simulink model "MAIN"  (R2023a)
settings: Solver=FixedStepDiscrete  StartTime=0.0  StopTime=10.0  FixedStep=1e-5  RelTol=1e-3
libraries: eeGeneralControl x2, simulink_extras x1
settings Model: Creator=james  LastModifiedBy=james
settings OptimizationCC: DefaultParameterBehavior=Inlined  UseDivisionForNetSlopeComputation=on  GainParamInheritBuiltInType=on  UseFloatMulNetSlope=on  InlineInvariantSignals=on  PassReuseOutputArgsAs=Individual arguments  ZeroExternalMemoryAtStartup=off  ZeroInternalMemoryAtStartup=off  NoFixptDivByZeroProtection=on  EfficientFloat2IntCast=on  LifeSpan=1  OptimizeBlockOrder=speed  DifferentSizesBufferReuse=on  EfficientTunableParamExpr=on
settings DebuggingCC: ParameterTunabilityLossMsg=error
settings HardwareCC: ProdBitPerPointer=32  ProdBitPerSizeT=32  ProdBitPerPtrDiffT=32  ProdLargestAtomicInteger=Long  ProdLargestAtomicFloat=Double  ProdWordSize=32  ProdLongLongMode=on  ProdHWDeviceType=ARM Compatible->ARM Cortex-M
settings SFSimCC: MATLABDynamicMemAlloc=off
settings RTWCC: Description=Embedded Coder  SystemTargetFile=ert.tlc  GenCodeOnly=on  TemplateMakefile=ert_default_tmf  GenerateReport=on  LaunchReport=on  GenerateCodeReplacementReport=on
settings CodeAppCC: ForceParamTrailComments=on  IgnoreCustomStorageClasses=off  OperatorAnnotations=on  SimulinkDataObjDesc=on  SFDataObjDesc=on  CustomSymbolStrGlobalVar=rt$N$M  CustomSymbolStrType=$N$M  CustomSymbolStrFcn=$N$M$F  CustomSymbolStrMacro=$N$M  InsertBlockDesc=on
settings ERTTargetCC: TargetLangStandard=C99 (ISO)  CodeReplacementLibrary=ARM Cortex-M  GenerateSampleERTMain=on  IncludeMdlTerminateFcn=off  CombineSignalStateStructs=on  SuppressErrorStatus=on  SupportAbsoluteTime=off  SupportNonFinite=off  SupportComplex=off  InlinedParameterPlacement=NonHierarchical  ERTCustomFileTemplate=example_file_process.tlc  ERTFilePackagingFormat=CompactWithDataFile

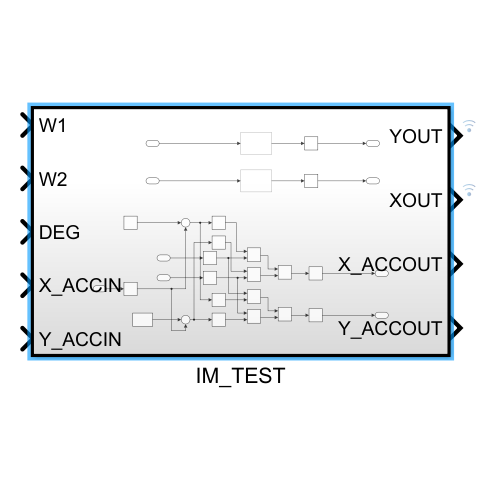
[thumbnail: Simulink's stored preview of the top-level diagram]
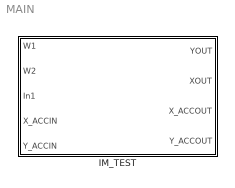
== system MAIN ==
  IM_TEST : Subsystem  TreatAsAtomicUnit=on
      settings: RTWSystemCode=Nonreusable function

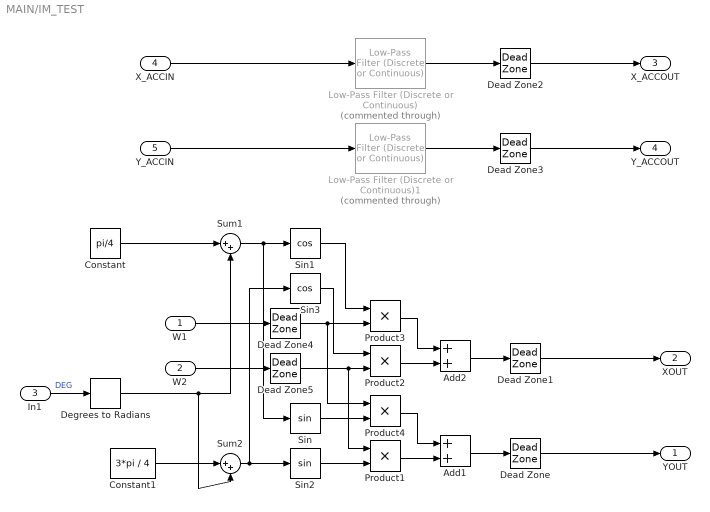
== system MAIN/IM_TEST ==
  W1 : Inport  OutDataTypeStr=single  LockScale=on
  W2 : Inport  Port=2  OutDataTypeStr=single  LockScale=on
  In1 : Inport  Port=3  OutDataTypeStr=single
  X_ACCIN : Inport  Port=4
  Y_ACCIN : Inport  Port=5
  Add1 : Sum
  Add2 : Sum
  Constant : Constant  Value=pi/4  OutDataTypeStr=single  LockScale=on
  Constant1 : Constant  Value=3*pi / 4  OutDataTypeStr=single  LockScale=on
  Dead Zone : DeadZone  LowerValue=-0.0005  UpperValue=0.00005
  Dead Zone1 : DeadZone  LowerValue=-0.0005  UpperValue=0.00005
  Dead Zone2 : DeadZone  LowerValue=-0.1  UpperValue=0.1
  Dead Zone3 : DeadZone  LowerValue=-0.1  UpperValue=0.1
  Dead Zone4 : DeadZone  LowerValue=-30  UpperValue=30
  Dead Zone5 : DeadZone  LowerValue=-30  UpperValue=30
  Degrees to Radians : simulink_extras/Transformations/Degrees to Radians
  Low-Pass Filter (Discrete or Continuous) : eeGeneralControl/Low-Pass Filter (Discrete or Continuous)  Commented=through  K=1  T=0.1  B=inf  A=-inf  init_option=Inherited from block input  x0=0  Ts=-1
  Low-Pass Filter (Discrete or Continuous)1 : eeGeneralControl/Low-Pass Filter (Discrete or Continuous)  Commented=through  K=1  T=0.1  B=inf  A=-inf  init_option=Inherited from block input  x0=0  Ts=-1
  Product{1..4} (4 alike) : Product
  Sin : Trigonometry  ApproximationMethod=Lookup
  Sin1 : Trigonometry  Operator=cos  ApproximationMethod=Lookup
  Sin2 : Trigonometry  ApproximationMethod=Lookup  OutputSignalType=real
  Sin3 : Trigonometry  Operator=cos  ApproximationMethod=Lookup
  Sum1 : Sum  Inputs=|++  AccumDataTypeStr=single
  Sum2 : Sum  Inputs=|++  AccumDataTypeStr=single
  YOUT : Outport
  XOUT : Outport  Port=2
  X_ACCOUT : Outport  Port=3
  Y_ACCOUT : Outport  Port=4
  wires:
  Constant1/1 -> Sum2/1
  In1/1 -> Degrees to Radians/1  "DEG"
  Sum2/1 -> Sin2/1, Sin3/1
  Constant/1 -> Sum1/1
  Degrees to Radians/1 -> Sum1/2, Sum2/2
  Sum1/1 -> Sin1/1, Sin/1
  Sin1/1 -> Product3/1
  Sin3/1 -> Product2/1
  W1/1 -> Dead Zone4/1
  W2/1 -> Dead Zone5/1
  Sin2/1 -> Product1/2
  Sin/1 -> Product4/2
  Product3/1 -> Add2/1
  Product2/1 -> Add2/2
  Product4/1 -> Add1/1
  Product1/1 -> Add1/2
  Add2/1 -> Dead Zone1/1
  Add1/1 -> Dead Zone/1
  Dead Zone1/1 -> XOUT/1
  Dead Zone/1 -> YOUT/1
  X_ACCIN/1 -> Low-Pass Filter (Discrete or Continuous)/1
  Y_ACCIN/1 -> Low-Pass Filter (Discrete or Continuous)1/1
  Low-Pass Filter (Discrete or Continuous)/1 -> Dead Zone2/1
  Low-Pass Filter (Discrete or Continuous)1/1 -> Dead Zone3/1
  Dead Zone2/1 -> X_ACCOUT/1
  Dead Zone3/1 -> Y_ACCOUT/1
  Dead Zone4/1 -> Product3/2, Product4/1
  Dead Zone5/1 -> Product1/1, Product2/2
